simulink model "kinovaMicoSimscapeModel"  (R2021b)
settings: Solver=VariableStepAuto  StartTime=0.0  StopTime=0.3  FixedStep=0.01  RelTol=1e-3
PostLoadFcn:
  | micoRigidBodyTreeCreation;
  | IC=deg2rad([-90,180,180,0,0,0]);
  | interactiveHomePosition=deg2rad([-90 90 177.5 90 0 0]');
  | load("./KinovaMicoSimscapeVariantConfigurations.mat");
values from neighbouring files (symbols this model uses):
  micoCandlePosition = deg2rad([0,180,180,0,0,0])    [KinovaMicoSimscapeInitializeScript.m]    (also in generatingRandomTrajectory.m)
  ViaPointsTaskSpace = [ViaPointsTaskSpace;[[pi;0;pi],[pi;0;pi],[pi;0;pi],[pi;0;pi],[0;0;0],[0;0;0],[pi;0;pi]]]    [KinovaMicoSimscapeInitializeScript.m]    (also in generatingRandomTrajectory.m = [ViaPointsTaskSpace;zeros(3,7)])
undefined symbols (not defined in the file or in its folder): Mico, ViaPointsJointSpace, X, Y, Z
libraries: sm_lib x26, nesl_utility x19, robotcorelib x4, robotmaniplib x3, pid_lib x2
(part 31 of 50)

== matlab function kinovaMicoSimscapeModel/Variant Subsystem/TaskSpaceController/HybridImpedanceVelocityControl/H_RNE ==
  data: q input; M output
function M = fcn(q)

q1 = q(1);
q2 = q(2);
q3 = q(3);
q4 = q(4);
q5 = q(5);
q6 = q(6);



M1_1 = 0.0019936*cos(q3 + q4 + q5) - 0.000030223*cos(2.0*q2 - 2.0*q3 + 2.0*q4 - 1.0*q5) - 0.00012374*cos(2.0*q3 - 2.0*q2 + 2.0*q4 + 2.0*q5) - 0.000013749*cos(2.0*q2 - 2.0*q3 - 2.0*q4 + 2.0*q5) - 0.000013749*cos(2.0*q2 - 2.0*q3 + 2.0*q4 - 2.0*q5) - 0.00012374*cos(2.0*q2 - 2.0*q3 + 2.0*q4 + 2.0*q5) - 0.000095258*cos(2.0*q2 - 2.0*q3 - 1.0*q4 + 2.0*q5) - 0.0019936*cos(q3 - 2.0*q2 + q4 + q5) + 0.0085823*cos(q3 - 1.0*q4) - 0.002302*cos(q3 - 1.0*q5) - 0.000064163*cos(q4 - 1.0*q5) - 0.00018134*cos(2.0*q4 + q5) - 0.0085823*cos(2.0*q2 - 1.0*q3 + q4) - 0.005111*cos(2.0*q3 - 2.0*q2 + q4) + 0.002302*cos(2.0*q2 - 1.0*q3 + q5) + 0.005111*cos(2.0*q2 - 2.0*q3 + q4) - 0.0014978*cos(2.0*q3 - 2.0*q2 + q5) - 0.0014978*cos(2.0*q2 - 2.0*q3 + q5) - 0.00066454*cos(2.0*q2 - 1.0*q3 + q4 - 1.0*q5) + 0.00066454*cos(2.0*q2 - 1.0*q3 - 1.0*q4 + q5) + 0.00051961*cos(2.0*q2 - 2.0*q3 + q4 - 1.0*q5) - 0.00051961*cos(2.0*q2 - 2.0*q3 - 1.0*q4 + q5) + 0.00028577*cos(2.0*q3 - 2.0*q2 + q4 + 2.0*q5) + 0.000090668*cos(2.0*q3 - 2.0*q2 + 2.0*q4 + q5) + 0.000095258*cos(2.0*q2 - 2.0*q3 + q4 - 2.0*q5) - 0.00028577*cos(2.0*q2 - 2.0*q3 + q4 + 2.0*q5) - 0.000030223*cos(2.0*q2 - 2.0*q3 - 2.0*q4 + q5) + 0.000090668*cos(2.0*q2 - 2.0*q3 + 2.0*q4 + q5) - 0.074028*cos(2.0*q2) + 0.0010525*cos(2.0*q4) - 0.00016499*cos(2.0*q5) - 0.0085823*cos(q3 + q4) - 0.002302*cos(q3 + q5) + 0.00019249*cos(q4 + q5) + 0.0085823*cos(q3 - 2.0*q2 + q4) + 0.002302*cos(q3 - 2.0*q2 + q5) - 0.00066454*cos(q3 + q4 - 1.0*q5) + 0.00066454*cos(q3 - 1.0*q4 + q5) - 0.0019936*cos(q4 - 1.0*q3 + q5) + 0.0019936*cos(2.0*q2 - 1.0*q3 + q4 + q5) + 0.0011401*cos(2.0*q3 - 2.0*q2 + q4 + q5) - 0.0011401*cos(2.0*q2 - 2.0*q3 + q4 + q5) - 0.060795*cos(q3) - 0.00082864*cos(q4) + 0.002512*cos(q5) + 0.060795*cos(2.0*q2 - 1.0*q3) - 0.018292*cos(2.0*q2 - 2.0*q3) + 0.000060445*cos(2.0*q4 - 1.0*q5) + 0.000027498*cos(2.0*q4 - 2.0*q5) + 0.00024749*cos(2.0*q4 + 2.0*q5) - 0.00052627*cos(2.0*q3 - 2.0*q2 + 2.0*q4) - 0.00052627*cos(2.0*q2 - 2.0*q3 + 2.0*q4) - 0.00024749*cos(2.0*q3 - 2.0*q2 + 2.0*q5) - 0.00024749*cos(2.0*q2 - 2.0*q3 + 2.0*q5) + 0.10044;
 
M1_2 = 0.0011882*cos(q2 - 1.0*q3 + q4 + q5) - 0.0019936*cos(q2 + q4 + q5) + 0.0010919*cos(q3 - 1.0*q2 + q4 + q5) + 0.0010437*cos(q2 - 1.0*q3) + 0.0085823*cos(q2 - 1.0*q4) + 0.0010525*cos(q2 - 1.0*q3 + 2.0*q4) - 0.0010525*cos(q3 - 1.0*q2 + 2.0*q4) - 0.000095258*cos(q2 - 1.0*q3 - 1.0*q4 + 2.0*q5) + 0.000060445*cos(q2 - 1.0*q3 + 2.0*q4 - 1.0*q5) - 0.000027498*cos(q2 - 1.0*q3 - 2.0*q4 + 2.0*q5) + 0.000027498*cos(q2 - 1.0*q3 + 2.0*q4 - 2.0*q5) + 0.00024749*cos(q2 - 1.0*q3 + 2.0*q4 + 2.0*q5) - 0.00024749*cos(q3 - 1.0*q2 + 2.0*q4 + 2.0*q5) + 0.0085823*cos(q2 + q4) - 0.0053182*cos(q2 - 1.0*q3 + q4) - 0.0049038*cos(q3 - 1.0*q2 + q4) + 0.000055567*cos(q2 - 1.0*q3 + q5) + 0.000055567*cos(q3 - 1.0*q2 + q5) + 0.00066454*cos(q2 + q4 - 1.0*q5) + 0.00066454*cos(q2 - 1.0*q4 + q5) - 0.0019936*cos(q4 - 1.0*q2 + q5) - 0.00053566*cos(q2 - 1.0*q3 + q4 - 1.0*q5) - 0.00050357*cos(q2 - 1.0*q3 - 1.0*q4 + q5) - 0.000095258*cos(q2 - 1.0*q3 + q4 - 2.0*q5) + 0.00028577*cos(q2 - 1.0*q3 + q4 + 2.0*q5) - 0.000060445*cos(q2 - 1.0*q3 - 2.0*q4 + q5) - 0.00018134*cos(q2 - 1.0*q3 + 2.0*q4 + q5) + 0.00028577*cos(q3 - 1.0*q2 + q4 + 2.0*q5) + 0.00018134*cos(q3 - 1.0*q2 + 2.0*q4 + q5) - 0.0034131*cos(q2);
 
M1_3 = 0.0010525*cos(q3 - 1.0*q2 + 2.0*q4) - 0.0010919*cos(q3 - 1.0*q2 + q4 + q5) - 0.0010437*cos(q2 - 1.0*q3) - 0.0010525*cos(q2 - 1.0*q3 + 2.0*q4) - 0.0011882*cos(q2 - 1.0*q3 + q4 + q5) + 0.000095258*cos(q2 - 1.0*q3 - 1.0*q4 + 2.0*q5) - 0.000060445*cos(q2 - 1.0*q3 + 2.0*q4 - 1.0*q5) + 0.000027498*cos(q2 - 1.0*q3 - 2.0*q4 + 2.0*q5) - 0.000027498*cos(q2 - 1.0*q3 + 2.0*q4 - 2.0*q5) - 0.00024749*cos(q2 - 1.0*q3 + 2.0*q4 + 2.0*q5) + 0.00024749*cos(q3 - 1.0*q2 + 2.0*q4 + 2.0*q5) + 0.0053182*cos(q2 - 1.0*q3 + q4) + 0.0049038*cos(q3 - 1.0*q2 + q4) - 0.000055567*cos(q2 - 1.0*q3 + q5) - 0.000055567*cos(q3 - 1.0*q2 + q5) + 0.00053566*cos(q2 - 1.0*q3 + q4 - 1.0*q5) + 0.00050357*cos(q2 - 1.0*q3 - 1.0*q4 + q5) + 0.000095258*cos(q2 - 1.0*q3 + q4 - 2.0*q5) - 0.00028577*cos(q2 - 1.0*q3 + q4 + 2.0*q5) + 0.000060445*cos(q2 - 1.0*q3 - 2.0*q4 + q5) + 0.00018134*cos(q2 - 1.0*q3 + 2.0*q4 + q5) - 0.00028577*cos(q3 - 1.0*q2 + q4 + 2.0*q5) - 0.00018134*cos(q3 - 1.0*q2 + 2.0*q4 + q5);
 
M1_4 = 0.0019936*cos(q2 + q4 + q5) - 0.0010919*cos(q2 - 1.0*q3 + q4 + q5) + 0.0011882*cos(q3 - 1.0*q2 + q4 + q5) + 0.0068797*cos(q2 - 1.0*q3) + 0.0085823*cos(q2 - 1.0*q4) - 0.00032998*cos(q2 - 1.0*q3 + 2.0*q5) - 0.00032998*cos(q3 - 1.0*q2 + 2.0*q5) - 0.000095258*cos(q2 - 1.0*q3 - 1.0*q4 + 2.0*q5) - 0.0085823*cos(q2 + q4) + 0.0049038*cos(q2 - 1.0*q3 + q4) - 0.0053182*cos(q3 - 1.0*q2 + q4) - 0.00024178*cos(q2 - 1.0*q3 + q5) - 0.00024178*cos(q3 - 1.0*q2 + q5) - 0.00066454*cos(q2 + q4 - 1.0*q5) + 0.00066454*cos(q2 - 1.0*q4 + q5) - 0.0019936*cos(q4 - 1.0*q2 + q5) + 0.00050357*cos(q2 - 1.0*q3 + q4 - 1.0*q5) - 0.00053566*cos(q2 - 1.0*q3 - 1.0*q4 + q5) + 0.000095258*cos(q2 - 1.0*q3 + q4 - 2.0*q5) - 0.00028577*cos(q2 - 1.0*q3 + q4 + 2.0*q5) + 0.00028577*cos(q3 - 1.0*q2 + q4 + 2.0*q5);
 
M1_5 = 0.0019936*cos(q2 + q4 + q5) - 0.0013013*cos(q2 - 1.0*q3 + q4 + q5) + 0.0013976*cos(q3 - 1.0*q2 + q4 + q5) + 0.0012634*cos(q2 - 1.0*q3) - 0.0010941*cos(q2 - 1.0*q3 + q4) + 0.0010941*cos(q3 - 1.0*q2 + q4) - 0.00018621*cos(q2 - 1.0*q3 + q5) - 0.00029735*cos(q3 - 1.0*q2 + q5) + 0.00066454*cos(q2 + q4 - 1.0*q5) - 0.00066454*cos(q2 - 1.0*q4 + q5) - 0.0019936*cos(q4 - 1.0*q2 + q5) - 0.00029419*cos(q2 - 1.0*q3 + q4 - 1.0*q5) + 0.00032627*cos(q2 - 1.0*q3 - 1.0*q4 + q5);
 
M1_6 = 0.00020265*cos(q2 - 1.0*q3 + q4 + q5) - 0.00020265*cos(q3 - 1.0*q2 + q4 + q5) + 0.000156*cos(q2 - 1.0*q3) - 0.0001351*cos(q2 - 1.0*q3 + q4) + 0.0001351*cos(q3 - 1.0*q2 + q4) + 0.000234*cos(q2 - 1.0*q3 + q5) + 0.000234*cos(q3 - 1.0*q2 + q5) - 0.00006755*cos(q2 - 1.0*q3 + q4 - 1.0*q5) + 0.00006755*cos(q2 - 1.0*q3 - 1.0*q4 + q5);
 
M2_1 = 0.0010437*cos(q2)*cos(q3) - 0.0034131*cos(q2) + 0.017165*cos(q2)*cos(q4) + 0.0010437*sin(q2)*sin(q3) + 0.0021051*sin(2.0*q4)*cos(q2)*sin(q3) - 0.0021051*sin(2.0*q4)*cos(q3)*sin(q2) - 0.010222*cos(q2)*cos(q3)*cos(q4) + 0.00011113*cos(q2)*cos(q3)*cos(q5) - 0.0026582*cos(q2)*cos(q4)*cos(q5) - 0.00041432*cos(q2)*sin(q3)*sin(q4) + 0.00041432*cos(q3)*sin(q2)*sin(q4) - 0.010222*cos(q4)*sin(q2)*sin(q3) + 0.00011113*cos(q5)*sin(q2)*sin(q3) + 0.0053164*cos(q2)*sin(q4)*sin(q5) + 0.00043998*cos(2.0*q4)*sin(2.0*q5)*cos(q2)*sin(q3) - 0.00043998*cos(2.0*q4)*sin(2.0*q5)*cos(q3)*sin(q2) + 0.00054997*cos(2.0*q5)*sin(2.0*q4)*cos(q2)*sin(q3) - 0.00054997*cos(2.0*q5)*sin(2.0*q4)*cos(q3)*sin(q2) + 0.00038103*cos(2.0*q5)*cos(q2)*cos(q3)*cos(q4) - 0.00048356*cos(2.0*q4)*cos(q2)*sin(q3)*sin(q5) + 0.00048356*cos(2.0*q4)*cos(q3)*sin(q2)*sin(q5) + 0.00038103*cos(2.0*q5)*cos(q4)*sin(q2)*sin(q3) - 0.00024178*sin(2.0*q4)*cos(q2)*cos(q5)*sin(q3) + 0.00024178*sin(2.0*q4)*cos(q3)*cos(q5)*sin(q2) - 0.00076206*sin(2.0*q5)*cos(q2)*cos(q3)*sin(q4) - 0.00076206*sin(2.0*q5)*sin(q2)*sin(q3)*sin(q4) + 0.0012409*cos(q2)*cos(q3)*cos(q4)*cos(q5) - 0.0033194*cos(q2)*cos(q3)*sin(q4)*sin(q5) + 0.00012833*cos(q2)*cos(q4)*sin(q3)*sin(q5) + 0.000064163*cos(q2)*cos(q5)*sin(q3)*sin(q4) - 0.00012833*cos(q3)*cos(q4)*sin(q2)*sin(q5) - 0.000064163*cos(q3)*cos(q5)*sin(q2)*sin(q4) + 0.0012409*cos(q4)*cos(q5)*sin(q2)*sin(q3) - 0.0033194*sin(q2)*sin(q3)*sin(q4)*sin(q5);
 
M2_2 = 0.00032998*cos(2.0*q5) - 0.0021051*cos(2.0*q4) - 0.12159*cos(q3) + 0.0055075*cos(q5) - 0.0092082*cos(q3)*cos(q5) + 0.034329*sin(q3)*sin(q4) - 0.00054997*cos(2.0*q4)*cos(2.0*q5) + 0.00043998*sin(2.0*q4)*sin(2.0*q5) + 0.00024178*cos(2.0*q4)*cos(q5) - 0.00048356*sin(2.0*q4)*sin(q5) - 0.010633*cos(q4)*sin(q3)*sin(q5) - 0.0053164*cos(q5)*sin(q3)*sin(q4) + 0.19203;
 
M2_3 = 0.0021051*cos(2.0*q4) - 0.00032998*cos(2.0*q5) + 0.060795*cos(q3) - 0.0055075*cos(q5) + 0.0046041*cos(q3)*cos(q5) - 0.017165*sin(q3)*sin(q4) + 0.00054997*cos(2.0*q4)*cos(2.0*q5) - 0.00043998*sin(2.0*q4)*sin(2.0*q5) - 0.00024178*cos(2.0*q4)*cos(q5) + 0.00048356*sin(2.0*q4)*sin(q5) + 0.0053164*cos(q4)*sin(q3)*sin(q5) + 0.0026582*cos(q5)*sin(q3)*sin(q4) - 0.043584;
 
M2_4 = 0.017165*cos(q3)*cos(q4) - 0.010222*cos(q4) + 0.0012409*cos(q4)*cos(q5) - 0.0033194*sin(q4)*sin(q5) + 0.00038103*cos(2.0*q5)*cos(q4) - 0.00076206*sin(2.0*q5)*sin(q4) - 0.0026582*cos(q3)*cos(q4)*cos(q5) + 0.0053164*cos(q3)*sin(q4)*sin(q5);
 
M2_5 = 0.0021882*cos(q4) + 0.0033194*cos(q4)*cos(q5) - 0.0046041*sin(q3)*sin(q5) - 0.0020785*sin(q4)*sin(q5) - 0.0053164*cos(q3)*cos(q4)*cos(q5) + 0.0026582*cos(q3)*sin(q4)*sin(q5);
 
M2_6 = 0.0002702*cos(q4) - 0.0002702*cos(q4)*cos(q5) + 0.0005404*sin(q4)*sin(q5);
 
M3_1 = 0.0021051*sin(2.0*q4)*cos(q3)*sin(q2) - 0.0010437*sin(q2)*sin(q3) - 0.0021051*sin(2.0*q4)*cos(q2)*sin(q3) - 0.0010437*cos(q2)*cos(q3) + 0.010222*cos(q2)*cos(q3)*cos(q4) - 0.00011113*cos(q2)*cos(q3)*cos(q5) + 0.00041432*cos(q2)*sin(q3)*sin(q4) - 0.00041432*cos(q3)*sin(q2)*sin(q4) + 0.010222*cos(q4)*sin(q2)*sin(q3) - 0.00011113*cos(q5)*sin(q2)*sin(q3) - 0.00043998*cos(2.0*q4)*sin(2.0*q5)*cos(q2)*sin(q3) + 0.00043998*cos(2.0*q4)*sin(2.0*q5)*cos(q3)*sin(q2) - 0.00054997*cos(2.0*q5)*sin(2.0*q4)*cos(q2)*sin(q3) + 0.00054997*cos(2.0*q5)*sin(2.0*q4)*cos(q3)*sin(q2) - 0.00038103*cos(2.0*q5)*cos(q2)*cos(q3)*cos(q4) + 0.00048356*cos(2.0*q4)*cos(q2)*sin(q3)*sin(q5) - 0.00048356*cos(2.0*q4)*cos(q3)*sin(q2)*sin(q5) - 0.00038103*cos(2.0*q5)*cos(q4)*sin(q2)*sin(q3) + 0.00024178*sin(2.0*q4)*cos(q2)*cos(q5)*sin(q3) - 0.00024178*sin(2.0*q4)*cos(q3)*cos(q5)*sin(q2) + 0.00076206*sin(2.0*q5)*cos(q2)*cos(q3)*sin(q4) + 0.00076206*sin(2.0*q5)*sin(q2)*sin(q3)*sin(q4) - 0.0012409*cos(q2)*cos(q3)*cos(q4)*cos(q5) + 0.0033194*cos(q2)*cos(q3)*sin(q4)*sin(q5) - 0.00012833*cos(q2)*cos(q4)*sin(q3)*sin(q5) - 0.000064163*cos(q2)*cos(q5)*sin(q3)*sin(q4) + 0.00012833*cos(q3)*cos(q4)*sin(q2)*sin(q5) + 0.000064163*cos(q3)*cos(q5)*sin(q2)*sin(q4) - 0.0012409*cos(q4)*cos(q5)*sin(q2)*sin(q3) + 0.0033194*sin(q2)*sin(q3)*sin(q4)*sin(q5);
 
M3_2 = 0.0021051*cos(2.0*q4) - 0.00032998*cos(2.0*q5) + 0.060795*cos(q3) - 0.0055075*cos(q5) + 0.0046041*cos(q3)*cos(q5) - 0.017165*sin(q3)*sin(q4) + 0.00054997*cos(2.0*q4)*cos(2.0*q5) - 0.00043998*sin(2.0*q4)*sin(2.0*q5) - 0.00024178*cos(2.0*q4)*cos(q5) + 0.00048356*sin(2.0*q4)*sin(q5) + 0.0053164*cos(q4)*sin(q3)*sin(q5) + 0.0026582*cos(q5)*sin(q3)*sin(q4) - 0.043584;
 
M3_3 = 0.00032998*cos(2.0*q5) - 0.0021051*cos(2.0*q4) + 0.0055075*cos(q5) - 0.00054997*cos(2.0*q4)*cos(2.0*q5) + 0.00043998*sin(2.0*q4)*sin(2.0*q5) + 0.00024178*cos(2.0*q4)*cos(q5) - 0.00048356*sin(2.0*q4)*sin(q5) + 0.043584;
 
M3_4 = 0.010222*cos(q4) - 0.0012409*cos(q4)*cos(q5) + 0.0033194*sin(q4)*sin(q5) - 0.00038103*cos(2.0*q5)*cos(q4) + 0.00076206*sin(2.0*q5)*sin(q4);
 
M3_5 = 0.0020785*sin(q4)*sin(q5) - 0.0033194*cos(q4)*cos(q5) - 0.0021882*cos(q4);
 
M3_6 = 0.0002702*cos(q4)*cos(q5) - 0.0002702*cos(q4) - 0.0005404*sin(q4)*sin(q5);
 
M4_1 = 0.0068797*cos(q2)*cos(q3) + 0.0068797*sin(q2)*sin(q3) + 0.017165*sin(q2)*sin(q4) - 0.00065996*cos(2.0*q5)*cos(q2)*cos(q3) - 0.00065996*cos(2.0*q5)*sin(q2)*sin(q3) - 0.00041432*cos(q2)*cos(q3)*cos(q4) - 0.00048356*cos(q2)*cos(q3)*cos(q5) + 0.010222*cos(q2)*sin(q3)*sin(q4) - 0.010222*cos(q3)*sin(q2)*sin(q4) - 0.00041432*cos(q4)*sin(q2)*sin(q3) - 0.00048356*cos(q5)*sin(q2)*sin(q3) - 0.0053164*cos(q4)*sin(q2)*sin(q5) - 0.0026582*cos(q5)*sin(q2)*sin(q4) - 0.00038103*cos(2.0*q5)*cos(q2)*sin(q3)*sin(q4) + 0.00038103*cos(2.0*q5)*cos(q3)*sin(q2)*sin(q4) - 0.00076206*sin(2.0*q5)*cos(q2)*cos(q4)*sin(q3) + 0.00076206*sin(2.0*q5)*cos(q3)*cos(q4)*sin(q2) + 0.000064163*cos(q2)*cos(q3)*cos(q4)*cos(q5) - 0.00012833*cos(q2)*cos(q3)*sin(q4)*sin(q5) - 0.0033194*cos(q2)*cos(q4)*sin(q3)*sin(q5) - 0.0012409*cos(q2)*cos(q5)*sin(q3)*sin(q4) + 0.0033194*cos(q3)*cos(q4)*sin(q2)*sin(q5) + 0.0012409*cos(q3)*cos(q5)*sin(q2)*sin(q4) + 0.000064163*cos(q4)*cos(q5)*sin(q2)*sin(q3) - 0.00012833*sin(q2)*sin(q3)*sin(q4)*sin(q5);
 
M4_2 = 0.017165*cos(q3)*cos(q4) - 0.010222*cos(q4) + 0.0012409*cos(q4)*cos(q5) - 0.0033194*sin(q4)*sin(q5) + 0.00038103*cos(2.0*q5)*cos(q4) - 0.00076206*sin(2.0*q5)*sin(q4) - 0.0026582*cos(q3)*cos(q4)*cos(q5) + 0.0053164*cos(q3)*sin(q4)*sin(q5);
 
M4_3 = 0.010222*cos(q4) - 0.0012409*cos(q4)*cos(q5) + 0.0033194*sin(q4)*sin(q5) - 0.00038103*cos(2.0*q5)*cos(q4) + 0.00076206*sin(2.0*q5)*sin(q4);
 
M4_4 = 0.0068797 - 0.00048356*cos(q5) - 0.00065996*cos(2.0*q5);
 
M4_5 = 0.0012634 - 0.00048356*cos(q5);
 
M4_6 = 0.000468*cos(q5) + 0.000156;
 
M5_1 = 0.0012634*cos(q2)*cos(q3) + 0.0012634*sin(q2)*sin(q3) - 0.00048356*cos(q2)*cos(q3)*cos(q5) - 0.0021882*cos(q2)*sin(q3)*sin(q4) + 0.0021882*cos(q3)*sin(q2)*sin(q4) + 0.00011113*cos(q2)*sin(q3)*sin(q5) - 0.00011113*cos(q3)*sin(q2)*sin(q5) - 0.00048356*cos(q5)*sin(q2)*sin(q3) - 0.0026582*cos(q4)*sin(q2)*sin(q5) - 0.0053164*cos(q5)*sin(q2)*sin(q4) + 0.00012833*cos(q2)*cos(q3)*cos(q4)*cos(q5) - 0.000064163*cos(q2)*cos(q3)*sin(q4)*sin(q5) - 0.0020785*cos(q2)*cos(q4)*sin(q3)*sin(q5) - 0.0033194*cos(q2)*cos(q5)*sin(q3)*sin(q4) + 0.0020785*cos(q3)*cos(q4)*sin(q2)*sin(q5) + 0.0033194*cos(q3)*cos(q5)*sin(q2)*sin(q4) + 0.00012833*cos(q4)*cos(q5)*sin(q2)*sin(q3) - 0.000064163*sin(q2)*sin(q3)*sin(q4)*sin(q5);
 
M5_2 = 0.0021882*cos(q4) + 0.0033194*cos(q4)*cos(q5) - 0.0046041*sin(q3)*sin(q5) - 0.0020785*sin(q4)*sin(q5) - 0.0053164*cos(q3)*cos(q4)*cos(q5) + 0.0026582*cos(q3)*sin(q4)*sin(q5);
 
M5_3 = 0.0020785*sin(q4)*sin(q5) - 0.0033194*cos(q4)*cos(q5) - 0.0021882*cos(q4);
 
M5_4 = 0.0012634 - 0.00048356*cos(q5);
 
M5_5 = 0.0025267;
 
M5_6 = 0.000312;
 
M6_1 = 0.000156*cos(q2 - 1.0*q3) + 0.000468*cos(q2 - 1.0*q3)*cos(q5) + 0.0002702*sin(q2 - 1.0*q3)*sin(q4) - 0.0005404*sin(q2 - 1.0*q3)*cos(q4)*sin(q5) - 0.0002702*sin(q2 - 1.0*q3)*cos(q5)*sin(q4);
 
M6_2 = 0.0002702*cos(q4) - 0.0002702*cos(q4)*cos(q5) + 0.0005404*sin(q4)*sin(q5);
 
M6_3 = 0.0002702*cos(q4)*cos(q5) - 0.0002702*cos(q4) - 0.0005404*sin(q4)*sin(q5);
 
M6_4 = 0.000468*cos(q5) + 0.000156;
 
M6_5 = 0.000312;
 
M6_6 = 0.000624;
 
 
M =[M1_1, M1_2, M1_3, M1_4, M1_5, M1_6;
    M2_1, M2_2, M2_3, M2_4, M2_5, M2_6;
    M3_1, M3_2, M3_3, M3_4, M3_5, M3_6;
    M4_1, M4_2, M4_3, M4_4, M4_5, M4_6;
    M5_1, M5_2, M5_3, M5_4, M5_5, M5_6;
    M6_1, M6_2, M6_3, M6_4, M6_5, M6_6];
